simulink model "lab_sim_0"  (R2022b)
settings: Solver=VariableStepAuto  StartTime=0.0  StopTime=100  MaxStep=1e-3  MinStep=1e-4  RelTol=1e-4
settings Model: Creator=yeyi5  LastModifiedBy=yeyi5
settings DataIOCC: ReturnWorkspaceOutputs=off

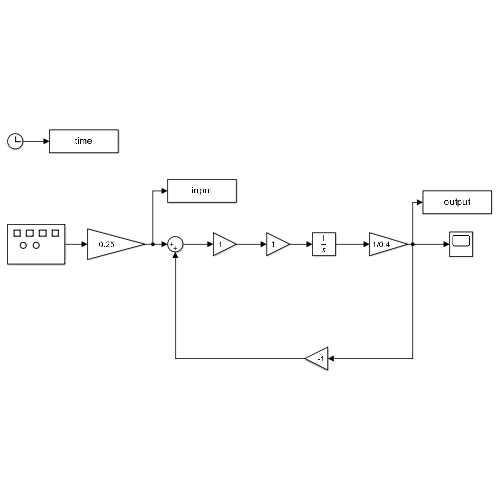
[thumbnail: Simulink's stored preview of the top-level diagram]
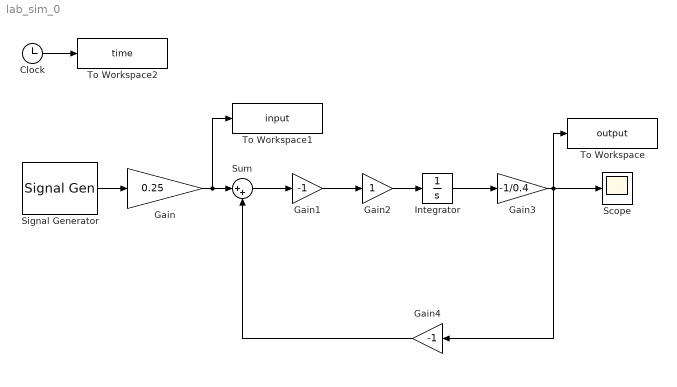
== system lab_sim_0 ==
  Clock : Clock
  Gain : Gain  Gain=0.25
  Gain1 : Gain  Gain=-1
  Gain2 : Gain
  Gain3 : Gain  Gain=-1/0.4
  Gain4 : Gain  Gain=-1
  Integrator : Integrator
  Scope : Scope
  Signal Generator : SignalGenerator  WaveForm=square  Amplitude=10  Frequency=0.1
  Sum : Sum  Inputs=|++
  To Workspace : ToWorkspace  VariableName=output  SampleTime=-1
  To Workspace1 : ToWorkspace  VariableName=input  SampleTime=-1
  To Workspace2 : ToWorkspace  VariableName=time  SampleTime=-1
  wires:
  Signal Generator/1 -> Gain/1
  Gain/1 -> To Workspace1/1, Sum/1
  Sum/1 -> Gain1/1
  Gain1/1 -> Gain2/1
  Gain3/1 -> Gain4/1, To Workspace/1, Scope/1
  Gain4/1 -> Sum/2
  Gain2/1 -> Integrator/1
  Integrator/1 -> Gain3/1
  Clock/1 -> To Workspace2/1
